simulink model "lab2part3"  (R2023a)
settings: Solver=ode45  StartTime=0.0  StopTime=3  MaxStep=.001  RelTol=1e-3
values from neighbouring files (symbols this model uses):
  a = 50    [lab2part1plot.m]    (also in lab2part2plot.m = as(i); lab2part3plot.m = as(i))
  A = [-6 -25; 1 0]    [lab2part1plot.m]    (also in lab2part2plot.m; lab2part3plot.m)
  B = [25; 0]    [lab2part1plot.m]    (also in lab2part2plot.m; lab2part3plot.m)
  C = [1 0; 0 1]    [lab2part1plot.m]    (also in lab2part2plot.m; lab2part3plot.m)
  D = [0; 0]    [lab2part1plot.m]    (also in lab2part2plot.m; lab2part3plot.m)
  zeta = 0.6    [lab2part1plot.m]    (also in lab2part2plot.m; lab2part3plot.m)
settings Model: Creator=rar4  LastModifiedBy=rar4

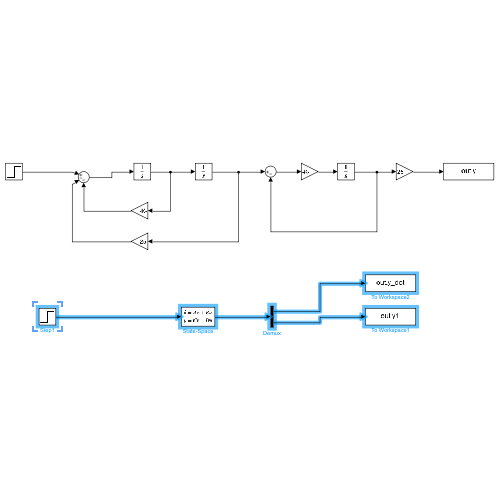
[thumbnail: Simulink's stored preview of the top-level diagram]
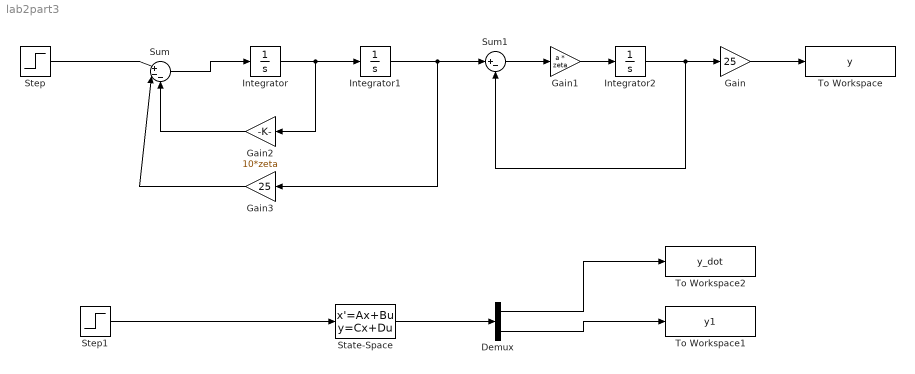
== system lab2part3 ==
  Demux : Demux  Outputs=2
  Gain : Gain  Gain=25
  Gain1 : Gain  Gain=a * zeta
  Gain2 : Gain  Gain=10*zeta
  Gain3 : Gain  Gain=25
  Integrator : Integrator
  Integrator1 : Integrator
  Integrator2 : Integrator
  State-Space : StateSpace  A=A  B=B  C=C  D=D  InitialCondition=0
  Step : Step  Time=0  SampleTime=0
  Step1 : Step  Time=0  SampleTime=0
  Sum : Sum  Inputs=|+--
  Sum1 : Sum  Inputs=|+-
  To Workspace : ToWorkspace  VariableName=y  SampleTime=-1
  To Workspace1 : ToWorkspace  VariableName=y1  SampleTime=-1
  To Workspace2 : ToWorkspace  VariableName=y_dot  SampleTime=-1
  wires:
  Integrator1/1 -> Sum1/1, Gain3/1
  Integrator/1 -> Gain2/1, Integrator1/1
  Step1/1 -> State-Space/1
  State-Space/1 -> Demux/1
  Demux/1 -> To Workspace2/1
  Demux/2 -> To Workspace1/1
  Gain/1 -> To Workspace/1
  Integrator2/1 -> Sum1/2, Gain/1
  Sum/1 -> Integrator/1
  Gain2/1 -> Sum/3
  Step/1 -> Sum/1
  Gain3/1 -> Sum/2
  Gain1/1 -> Integrator2/1
  Sum1/1 -> Gain1/1
